simulink model "Transmission_Model"  (R2016b)
settings: Solver=FixedStepDiscrete  StartTime=0.0  StopTime=inf  FixedStep=0.01  RelTol=1e-3  EnableMultiTasking=on
settings Model: Creator=m01wolf  LastModifiedBy=bunver
settings DataIOCC: SaveFormat=StructureWithTime  SaveOutput=off  DSMLogging=off  VisualizeSimOutput=off  SaveTime=off  StateSaveName=Results  SignalLoggingName=Results
settings OptimizationCC: BlockReduction=off  ConditionallyExecuteInputs=off  LifeSpan=inf
settings DebuggingCC: AllowSymbolicDim=off  SFUnexpectedBacktrackingDiag=warning  SFNoUnconditionalDefaultTransitionDiag=warning  SFExecutionAtInitializationDiag=none
settings ModelReferenceCC: ModelReferenceNumInstancesAllowed=Single  PropagateSignalLabelsOutOfModel=off
settings GRTTargetCC: TargetLangStandard=C89/C90 (ANSI)
settings ConfigComp: CovMetricSettings=dw  CovHtmlReporting=on  CovSaveCumulativeToWorkspaceVar=on  CovSaveSingleToWorkspaceVar=on  CovExternalEMLEnable=off

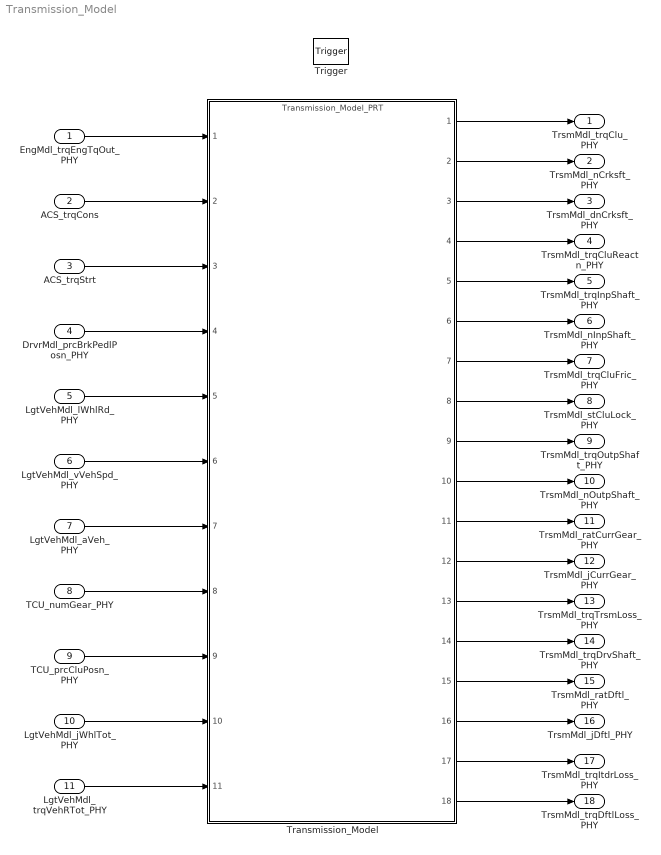
== system Transmission_Model ==
  EngMdl_trqEngTqOut_PHY : Inport
  ACS_trqCons : Inport  Port=2
  ACS_trqStrt : Inport  Port=3
  DrvrMdl_prcBrkPedlPosn_PHY : Inport  Port=4
  LgtVehMdl_lWhlRd_PHY : Inport  Port=5
  LgtVehMdl_vVehSpd_PHY : Inport  Port=6
  LgtVehMdl_aVeh_PHY : Inport  Port=7
  TCU_numGear_PHY : Inport  Port=8
  TCU_prcCluPosn_PHY : Inport  Port=9
  LgtVehMdl_jWhlTot_PHY : Inport  Port=10
  LgtVehMdl_trqVehRTot_PHY : Inport  Port=11
  Trigger : TriggerPort  TriggerType=function-call  VariantControl=Variant  PortDimensions=1
  Transmission_Model : ModelReference  ModelNameDialog=Transmission_Model_PRT.slxp  ModelReferenceVersion=1.202  CopyOfModelProtected=on
  TrsmMdl_trqClu_PHY : Outport
  TrsmMdl_nCrksft_PHY : Outport  Port=2
  TrsmMdl_dnCrksft_PHY : Outport  Port=3
  TrsmMdl_trqCluReactn_PHY : Outport  Port=4
  TrsmMdl_trqInpShaft_PHY : Outport  Port=5
  TrsmMdl_nInpShaft_PHY : Outport  Port=6
  TrsmMdl_trqCluFric_PHY : Outport  Port=7
  TrsmMdl_stCluLock_PHY : Outport  Port=8
  TrsmMdl_trqOutpShaft_PHY : Outport  Port=9
  TrsmMdl_nOutpShaft_PHY : Outport  Port=10
  TrsmMdl_ratCurrGear_PHY : Outport  Port=11
  TrsmMdl_jCurrGear_PHY : Outport  Port=12
  TrsmMdl_trqTrsmLoss_PHY : Outport  Port=13
  TrsmMdl_trqDrvShaft_PHY : Outport  Port=14
  TrsmMdl_ratDftl_PHY : Outport  Port=15
  TrsmMdl_jDftl_PHY : Outport  Port=16
  TrsmMdl_trqItdrLoss_PHY : Outport  Port=17
  TrsmMdl_trqDftlLoss_PHY : Outport  Port=18
  wires:
  ACS_trqStrt/1 -> Transmission_Model/3
  ACS_trqCons/1 -> Transmission_Model/2
  EngMdl_trqEngTqOut_PHY/1 -> Transmission_Model/1
  DrvrMdl_prcBrkPedlPosn_PHY/1 -> Transmission_Model/4
  LgtVehMdl_lWhlRd_PHY/1 -> Transmission_Model/5
  LgtVehMdl_vVehSpd_PHY/1 -> Transmission_Model/6
  LgtVehMdl_aVeh_PHY/1 -> Transmission_Model/7
  TCU_numGear_PHY/1 -> Transmission_Model/8
  TCU_prcCluPosn_PHY/1 -> Transmission_Model/9
  LgtVehMdl_jWhlTot_PHY/1 -> Transmission_Model/10
  LgtVehMdl_trqVehRTot_PHY/1 -> Transmission_Model/11
  Transmission_Model/5 -> TrsmMdl_trqInpShaft_PHY/1
  Transmission_Model/6 -> TrsmMdl_nInpShaft_PHY/1
  Transmission_Model/7 -> TrsmMdl_trqCluFric_PHY/1
  Transmission_Model/8 -> TrsmMdl_stCluLock_PHY/1
  Transmission_Model/9 -> TrsmMdl_trqOutpShaft_PHY/1
  Transmission_Model/10 -> TrsmMdl_nOutpShaft_PHY/1
  Transmission_Model/17 -> TrsmMdl_trqItdrLoss_PHY/1
  Transmission_Model/18 -> TrsmMdl_trqDftlLoss_PHY/1
  Transmission_Model/1 -> TrsmMdl_trqClu_PHY/1
  Transmission_Model/2 -> TrsmMdl_nCrksft_PHY/1
  Transmission_Model/3 -> TrsmMdl_dnCrksft_PHY/1
  Transmission_Model/4 -> TrsmMdl_trqCluReactn_PHY/1
  Transmission_Model/11 -> TrsmMdl_ratCurrGear_PHY/1
  Transmission_Model/12 -> TrsmMdl_jCurrGear_PHY/1
  Transmission_Model/13 -> TrsmMdl_trqTrsmLoss_PHY/1
  Transmission_Model/14 -> TrsmMdl_trqDrvShaft_PHY/1
  Transmission_Model/15 -> TrsmMdl_ratDftl_PHY/1
  Transmission_Model/16 -> TrsmMdl_jDftl_PHY/1
